simulink model "t2"  (R2022b)
settings: Solver=VariableStepAuto  StartTime=0.0  StopTime=1000  RelTol=1e-3
libraries: fuzblock x1
settings Model: Creator=10441  LastModifiedBy=mingh

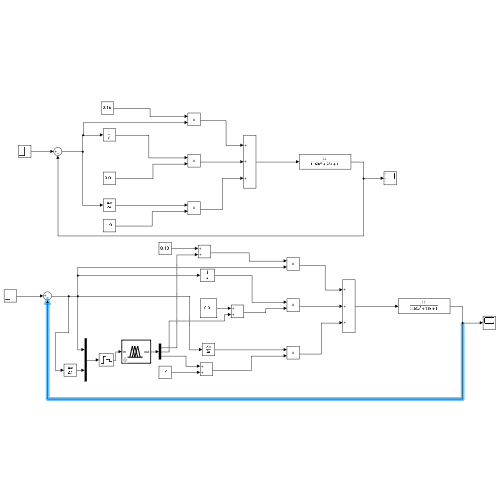
[thumbnail: Simulink's stored preview of the top-level diagram]
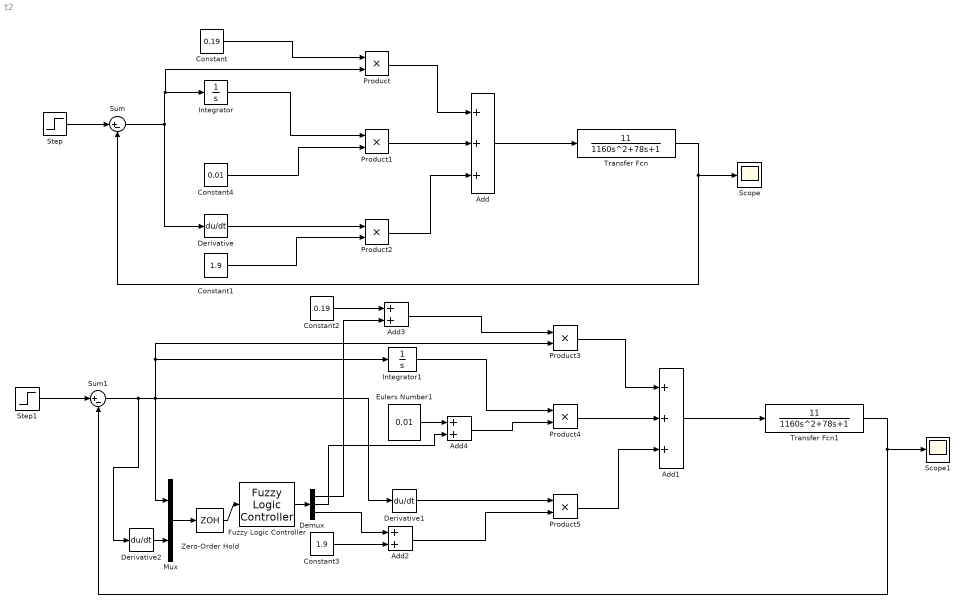
== system t2 ==
  Add : Sum  Inputs=+++
  Add1 : Sum  Inputs=+++
  Add2 : Sum
  Add3 : Sum
  Add4 : Sum
  Constant : Constant  Value=0.19
  Constant1 : Constant  Value=1.9
  Constant2 : Constant  Value=0.19
  Constant3 : Constant  Value=1.9
  Constant4 : Constant  Value=0.01
  Demux : Demux  Outputs=3
  Derivative : Derivative
  Derivative1 : Derivative
  Derivative2 : Derivative
  Eulers Number1 : Constant  Value=0.01  OutDataTypeStr=Inherit: Inherit via back propagation
  Fuzzy Logic Controller : fuzblock/Fuzzy Logic  Controller  FIS='t2.fis'  OutputSampleNumber=101  DataType=double  FuzzifiedInputs=off  RuleFiringStrengths=off  RuleOutputs=off  AggregatedOutputs=off  SimulateUsing=Interpreted execution  OutOfRangeInputValueMessage=warning  NoRuleFiredMessage=warning  EmptyOutputFuzzySetMessage=warning
  Integrator : Integrator
  Integrator1 : Integrator
  Mux : Mux  Inputs=2
  Product{,1..5} (6 alike) : Product
  Scope : Scope
  Scope1 : Scope
  Step : Step  SampleTime=0
  Step1 : Step  SampleTime=0
  Sum : Sum  Inputs=|+-
  Sum1 : Sum  Inputs=|+-
  Transfer Fcn : TransferFcn  Numerator=[11]  Denominator=[1160 78 1]
  Transfer Fcn1 : TransferFcn  Numerator=[11]  Denominator=[1160 78 1]
  Zero-Order Hold : ZeroOrderHold  SampleTime=-1
  wires:
  Step/1 -> Sum/1
  Constant/1 -> Product/1
  Sum/1 -> Product/2, Integrator/1, Derivative/1
  Integrator/1 -> Product1/1
  Constant4/1 -> Product1/2
  Derivative/1 -> Product2/1
  Constant1/1 -> Product2/2
  Transfer Fcn/1 -> Sum/2, Scope/1
  Product/1 -> Add/1
  Product1/1 -> Add/2
  Product2/1 -> Add/3
  Add/1 -> Transfer Fcn/1
  Add3/1 -> Product3/1
  Product4/1 -> Add1/2
  Add2/1 -> Product5/2
  Sum1/1 -> Derivative2/1, Mux/1, Product3/2, Integrator1/1, Derivative1/1
  Transfer Fcn1/1 -> Sum1/2, Scope1/1
  Product3/1 -> Add1/1
  Add1/1 -> Transfer Fcn1/1
  Integrator1/1 -> Product4/1
  Product5/1 -> Add1/3
  Derivative1/1 -> Product5/1
  Step1/1 -> Sum1/1
  Demux/3 -> Add2/1
  Constant3/1 -> Add2/2
  Add4/1 -> Product4/2
  Eulers Number1/1 -> Add4/1
  Constant2/1 -> Add3/1
  Demux/1 -> Add3/2
  Fuzzy Logic Controller/1 -> Demux/1
  Demux/2 -> Add4/2
  Derivative2/1 -> Mux/2
  Mux/1 -> Zero-Order Hold/1
  Zero-Order Hold/1 -> Fuzzy Logic Controller/1
